simulink model "hw2n_lawB"  (R2022b)
settings: Solver=VariableStepAuto  StartTime=0.0  StopTime=20.0  RelTol=1e-3
undefined symbols (not defined in the file or in its folder): orbit, sat
libraries: matrix_library x1
settings Model: Creator=gagandeepthapar  LastModifiedBy=gagandeepthapar

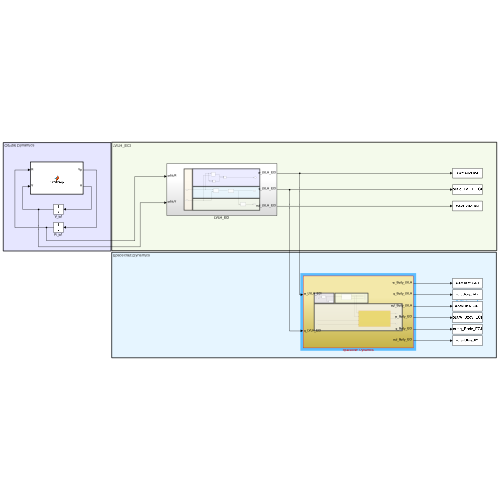
[thumbnail: Simulink's stored preview of the top-level diagram]
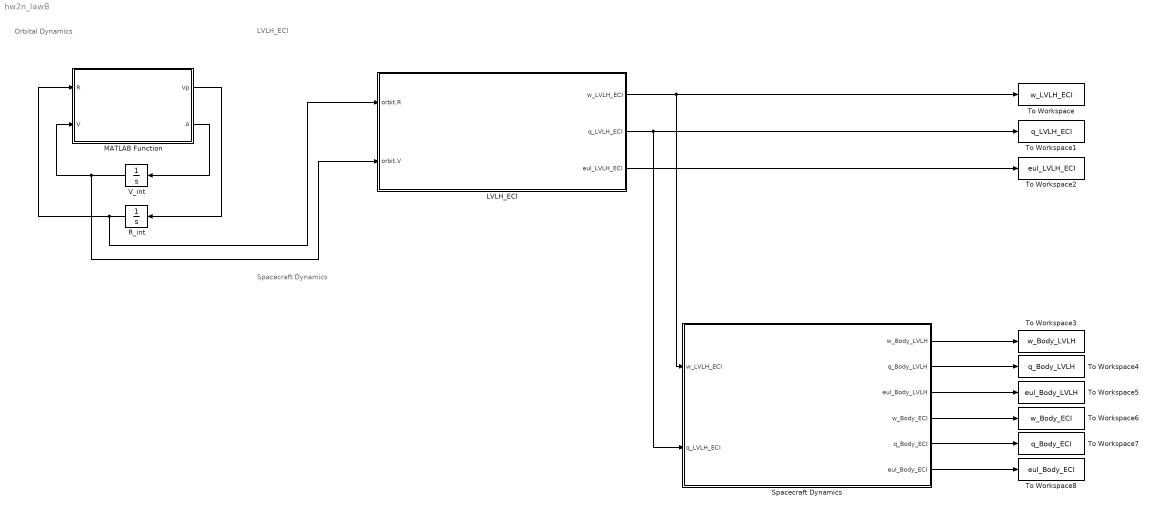
== system hw2n_lawB ==
  note: Spacecraft Dynamics
  note: LVLH_ECI
  note: Orbital Dynamics
  LVLH_ECI : Subsystem
  MATLAB Function : MATLAB Function  TreatAsAtomicUnit=on
  R_int : Integrator  InitialCondition=orbit.R0
  Spacecraft Dynamics : Subsystem
  To Workspace : ToWorkspace  VariableName=w_LVLH_ECI  SampleTime=-1
      settings: Save2DSignal=2-D array (concatenate along first dimension)
  To Workspace1 : ToWorkspace  VariableName=q_LVLH_ECI  SampleTime=-1
      settings: Save2DSignal=2-D array (concatenate along first dimension)
  To Workspace2 : ToWorkspace  VariableName=eul_LVLH_ECI  SampleTime=-1
      settings: Save2DSignal=2-D array (concatenate along first dimension)
  To Workspace3 : ToWorkspace  VariableName=w_Body_LVLH  SampleTime=-1
      settings: Save2DSignal=2-D array (concatenate along first dimension)
  To Workspace4 : ToWorkspace  VariableName=q_Body_LVLH  SampleTime=-1
      settings: Save2DSignal=2-D array (concatenate along first dimension)
  To Workspace5 : ToWorkspace  VariableName=eul_Body_LVLH  SampleTime=-1
      settings: Save2DSignal=2-D array (concatenate along first dimension)
  To Workspace6 : ToWorkspace  VariableName=w_Body_ECI  SampleTime=-1
      settings: Save2DSignal=2-D array (concatenate along first dimension)
  To Workspace7 : ToWorkspace  VariableName=q_Body_ECI  SampleTime=-1
      settings: Save2DSignal=2-D array (concatenate along first dimension)
  To Workspace8 : ToWorkspace  VariableName=eul_Body_ECI  SampleTime=-1
      settings: Save2DSignal=2-D array (concatenate along first dimension)
  V_int : Integrator  InitialCondition=orbit.V0
  wires:
  V_int/1 -> MATLAB Function/2(V), LVLH_ECI/2(orbit.V)
  MATLAB Function/2(A) -> V_int/1
  MATLAB Function/1(Vp) -> R_int/1
  R_int/1 -> MATLAB Function/1(R), LVLH_ECI/1(orbit.R)
  LVLH_ECI/3(eul_LVLH_ECI) -> To Workspace2/1
  LVLH_ECI/1(w_LVLH_ECI) -> To Workspace/1, Spacecraft Dynamics/1(w_LVLH_ECI)
  Spacecraft Dynamics/1(w_Body_LVLH) -> To Workspace3/1
  Spacecraft Dynamics/2(q_Body_LVLH) -> To Workspace4/1
  Spacecraft Dynamics/3(eul_Body_LVLH) -> To Workspace5/1
  Spacecraft Dynamics/5(q_Body_ECI) -> To Workspace7/1
  LVLH_ECI/2(q_LVLH_ECI) -> To Workspace1/1, Spacecraft Dynamics/2(q_LVLH_ECI)
  Spacecraft Dynamics/6(eul_Body_ECI) -> To Workspace8/1
  Spacecraft Dynamics/4(w_Body_ECI) -> To Workspace6/1

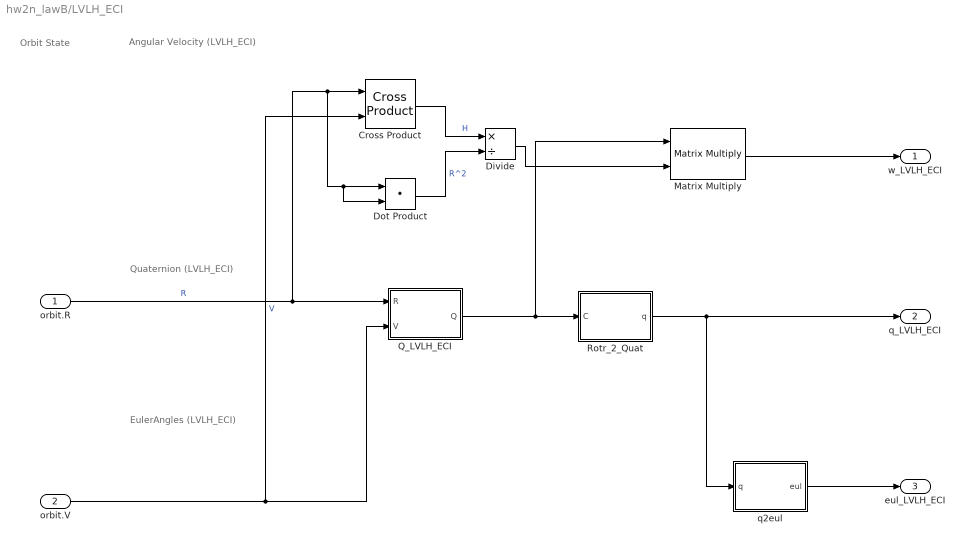
== system hw2n_lawB/LVLH_ECI ==
  note: EulerAngles (LVLH_ECI)
  note: Orbit State
  note: Quaternion (LVLH_ECI)
  note: Angular Velocity (LVLH_ECI)
  orbit.R : Inport
  orbit.V : Inport  Port=2
  Cross Product : matrix_library/Cross Product
  Divide : Product  Inputs=*/
  Dot Product : DotProduct  OutDataTypeStr=Inherit: Inherit via internal rule
  Matrix Multiply : Product  Multiplication=Matrix(*)
  Q_LVLH_ECI : MATLAB Function  TreatAsAtomicUnit=on
  Rotr_2_Quat : MATLAB Function  TreatAsAtomicUnit=on
  q2eul : MATLAB Function  TreatAsAtomicUnit=on
  w_LVLH_ECI : Outport
  q_LVLH_ECI : Outport  Port=2
  eul_LVLH_ECI : Outport  Port=3
  wires:
  orbit.R/1 -> Q_LVLH_ECI/1(R), Cross Product/1, Dot Product/1, Dot Product/2  "R"
  orbit.V/1 -> Cross Product/2, Q_LVLH_ECI/2(V)  "V"
  Q_LVLH_ECI/1(Q) -> Matrix Multiply/1, Rotr_2_Quat/1(C)
  Rotr_2_Quat/1(q) -> q2eul/1(q), q_LVLH_ECI/1
  q2eul/1(eul) -> eul_LVLH_ECI/1
  Cross Product/1 -> Divide/1  "H"
  Dot Product/1 -> Divide/2  "R^2"
  Divide/1 -> Matrix Multiply/2
  Matrix Multiply/1 -> w_LVLH_ECI/1

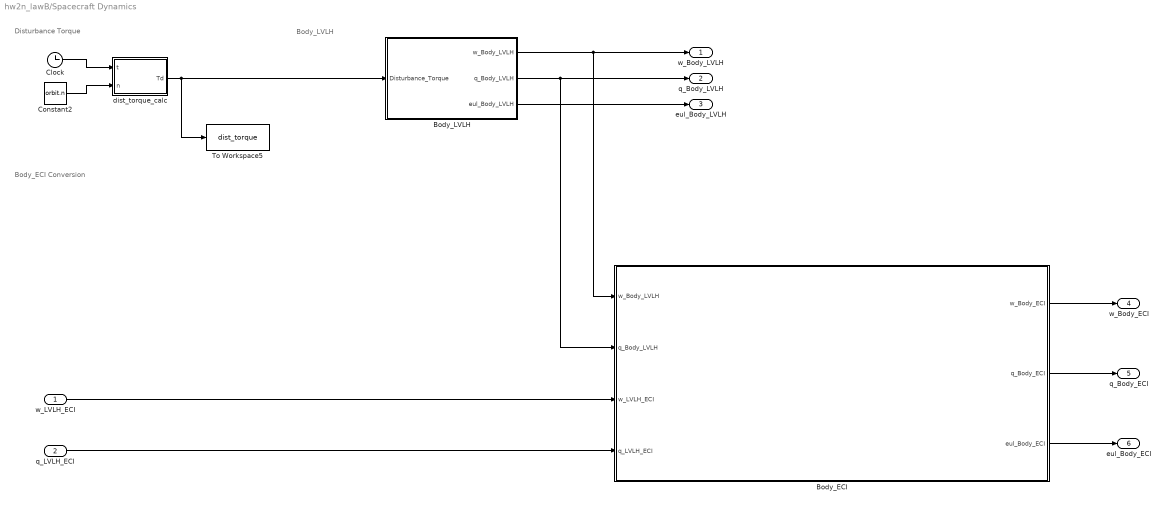
== system hw2n_lawB/Spacecraft Dynamics ==
  note: Body_ECI Conversion
  note: Body_LVLH
  note: Disturbance Torque
  w_LVLH_ECI : Inport
  q_LVLH_ECI : Inport  Port=2
  Body_ECI : Subsystem
  Body_LVLH : Subsystem
  Clock : Clock
  Constant2 : Constant  Value=orbit.n
  To Workspace5 : ToWorkspace  VariableName=dist_torque  SampleTime=-1
      settings: Save2DSignal=2-D array (concatenate along first dimension)
  dist_torque_calc : MATLAB Function  TreatAsAtomicUnit=on
  w_Body_LVLH : Outport
  q_Body_LVLH : Outport  Port=2
  eul_Body_LVLH : Outport  Port=3
  w_Body_ECI : Outport  Port=4
  q_Body_ECI : Outport  Port=5
  eul_Body_ECI : Outport  Port=6
  wires:
  Body_LVLH/1(w_Body_LVLH) -> w_Body_LVLH/1, Body_ECI/1(w_Body_LVLH)
  Body_LVLH/2(q_Body_LVLH) -> Body_ECI/2(q_Body_LVLH), q_Body_LVLH/1
  Body_LVLH/3(eul_Body_LVLH) -> eul_Body_LVLH/1
  Body_ECI/2(q_Body_ECI) -> q_Body_ECI/1
  Constant2/1 -> dist_torque_calc/2(n)
  dist_torque_calc/1(Td) -> Body_LVLH/1(Disturbance_Torque), To Workspace5/1
  Clock/1 -> dist_torque_calc/1(t)
  q_LVLH_ECI/1 -> Body_ECI/4(q_LVLH_ECI)
  w_LVLH_ECI/1 -> Body_ECI/3(w_LVLH_ECI)
  Body_ECI/1(w_Body_ECI) -> w_Body_ECI/1
  Body_ECI/3(eul_Body_ECI) -> eul_Body_ECI/1

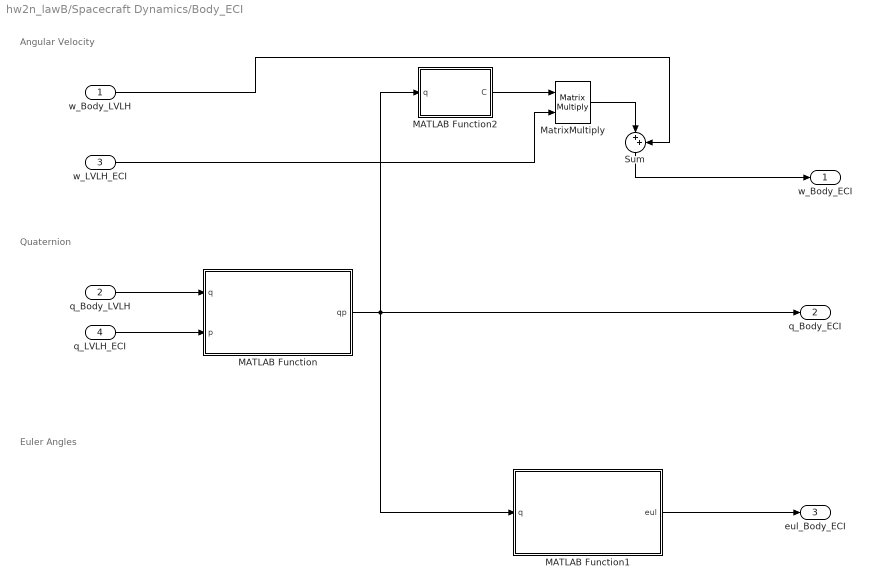
== system hw2n_lawB/Spacecraft Dynamics/Body_ECI ==
  note: Quaternion
  note: Euler Angles
  note: Angular Velocity
  w_Body_LVLH : Inport
  q_Body_LVLH : Inport  Port=2
  w_LVLH_ECI : Inport  Port=3
  q_LVLH_ECI : Inport  Port=4
  MATLAB Function : MATLAB Function  TreatAsAtomicUnit=on
  MATLAB Function1 : MATLAB Function  TreatAsAtomicUnit=on
  MATLAB Function2 : MATLAB Function  TreatAsAtomicUnit=on
  MatrixMultiply : Product  Multiplication=Matrix(*)
  Sum : Sum  Inputs=|++
  w_Body_ECI : Outport
  q_Body_ECI : Outport  Port=2
  eul_Body_ECI : Outport  Port=3
  wires:
  q_Body_LVLH/1 -> MATLAB Function/1(q)
  MATLAB Function/1(qp) -> MATLAB Function2/1(q), MATLAB Function1/1(q), q_Body_ECI/1
  q_LVLH_ECI/1 -> MATLAB Function/2(p)
  MATLAB Function1/1(eul) -> eul_Body_ECI/1
  Sum/1 -> w_Body_ECI/1
  MATLAB Function2/1(C) -> MatrixMultiply/1
  w_LVLH_ECI/1 -> MatrixMultiply/2
  MatrixMultiply/1 -> Sum/1
  w_Body_LVLH/1 -> Sum/2

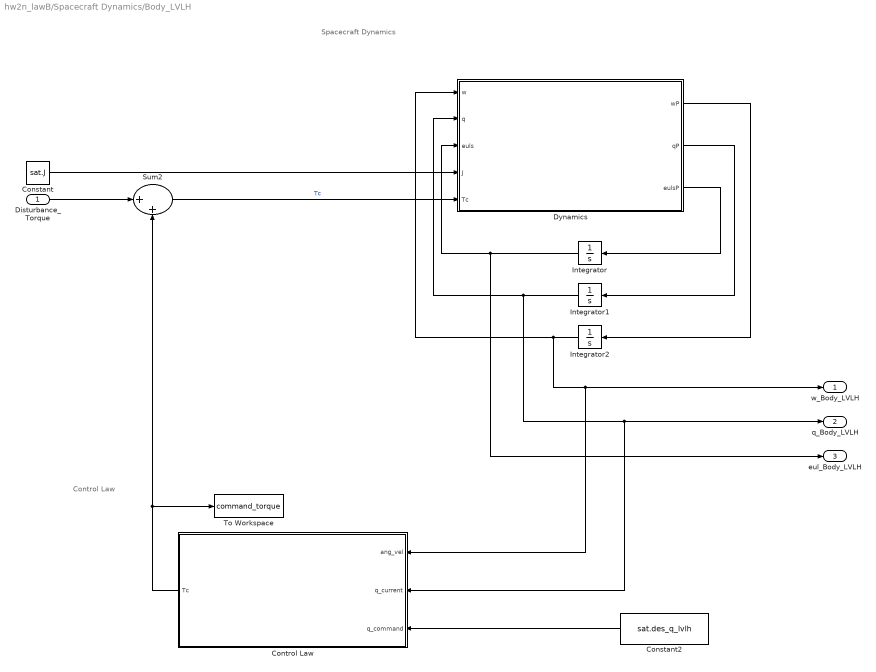
== system hw2n_lawB/Spacecraft Dynamics/Body_LVLH ==
  note: Spacecraft Dynamics
  note: Control Law
  Disturbance_Torque : Inport
  Constant : Constant  Value=sat.J
  Constant2 : Constant  Value=sat.des_q_lvlh
  Control Law : Subsystem
  Dynamics : MATLAB Function  TreatAsAtomicUnit=on
  Integrator : Integrator  InitialCondition=sat.euls0_lvlh
  Integrator1 : Integrator  InitialCondition=[sat.e0_lvlh;sat.n0_lvlh]
  Integrator2 : Integrator  InitialCondition=sat.w0_lvlh
  Sum2 : Sum  Inputs=|++
  To Workspace : ToWorkspace  VariableName=command_torque  SampleTime=-1
      settings: Save2DSignal=2-D array (concatenate along first dimension)
  w_Body_LVLH : Outport
  q_Body_LVLH : Outport  Port=2
  eul_Body_LVLH : Outport  Port=3
  wires:
  Dynamics/3(eulsP) -> Integrator/1
  Dynamics/2(qP) -> Integrator1/1
  Dynamics/1(wP) -> Integrator2/1
  Integrator/1 -> eul_Body_LVLH/1, Dynamics/3(euls)
  Integrator1/1 -> q_Body_LVLH/1, Control Law/2(q_current), Dynamics/2(q)
  Constant/1 -> Dynamics/4(J)
  Disturbance_Torque/1 -> Sum2/1
  Integrator2/1 -> w_Body_LVLH/1, Control Law/1(ang_vel), Dynamics/1(w)
  Sum2/1 -> Dynamics/5(Tc)  "Tc"
  Control Law/1(Tc) -> Sum2/2, To Workspace/1
  Constant2/1 -> Control Law/3(q_command)

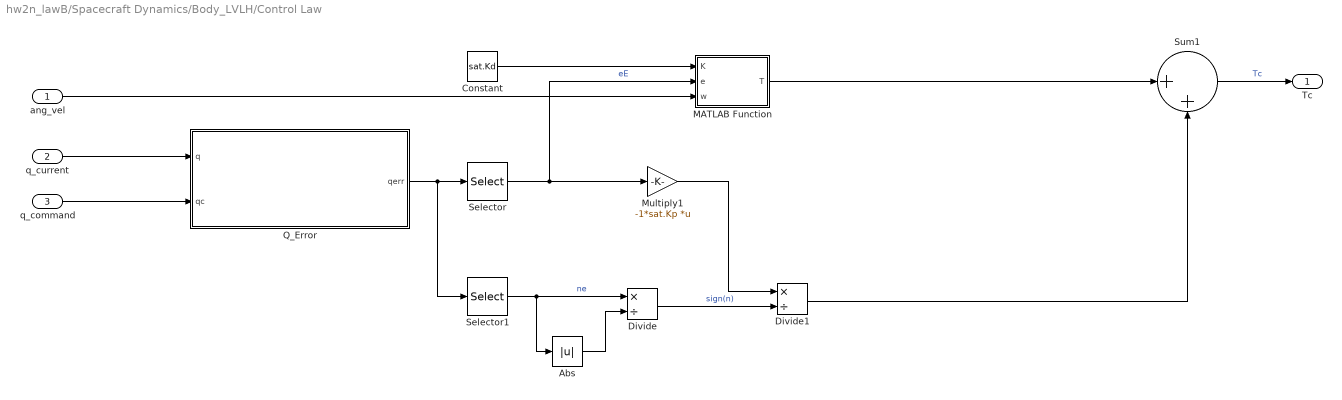
== system hw2n_lawB/Spacecraft Dynamics/Body_LVLH/Control Law ==
  ang_vel : Inport
  q_current : Inport  Port=2
  q_command : Inport  Port=3
  Abs : Abs  SaturateOnIntegerOverflow=off
  Constant : Constant  Value=sat.Kd
  Divide : Product  Inputs=*/
  Divide1 : Product  Inputs=*/
  MATLAB Function : MATLAB Function  TreatAsAtomicUnit=on
  Multiply1 : Gain  Gain=-1*sat.Kp  Multiplication=Matrix(K*u)
  Q_Error : MATLAB Function  TreatAsAtomicUnit=on
  Selector : Selector  InputPortWidth=4  IndexOptions=Index vector (dialog)  Indices=[1:3]  OutputSizes=1
  Selector1 : Selector  InputPortWidth=4  IndexOptions=Index vector (dialog)  Indices=[4]  OutputSizes=1
  Sum1 : Sum  Inputs=|++
  Tc : Outport
  wires:
  Sum1/1 -> Tc/1  "Tc"
  q_command/1 -> Q_Error/2(qc)
  Abs/1 -> Divide/2
  Selector/1 -> MATLAB Function/2(e), Multiply1/1  "eE"
  Divide/1 -> Divide1/2  "sign(n)"
  Selector1/1 -> Divide/1, Abs/1  "ne"
  q_current/1 -> Q_Error/1(q)
  Multiply1/1 -> Divide1/1
  Q_Error/1(qerr) -> Selector/1, Selector1/1
  Divide1/1 -> Sum1/2
  MATLAB Function/1(T) -> Sum1/1
  ang_vel/1 -> MATLAB Function/3(w)
  Constant/1 -> MATLAB Function/1(K)

== matlab function hw2n_lawB/LVLH_ECI/Q_LVLH_ECI ==
  data: R input; Q output; V input
function Q = fcn(R,V)


z = -1*R / norm(R);
y = -1 * cross(R,V) / norm(cross(R,V));

x = cross(y,z);

Q = [x,y,z]';

== matlab function hw2n_lawB/MATLAB Function ==
  data: R input; Vp output; V input; A output
function [Vp,A] = OrbitProp(R,V)

    mu = 398600;

    rad = norm(R);
    rx = R(1);
    ry = R(2);
    rz = R(3);

    ax = -mu*rx/rad^3;
    ay = -mu*ry/rad^3;
    az = -mu*rz/rad^3;

    Vp = [V(1);V(2);V(3)];
    A = [ax;ay;az];

end

== matlab function hw2n_lawB/LVLH_ECI/Rotr_2_Quat ==
  data: C input; q output
function q = fcn(C)

        e = zeros(3,1);
        n = 0.5 * sqrt(1 + trace(C));
        e(1) = 0.25 * (C(2,3) - C(3,2))/n;
        e(2) = 0.25 * (C(3,1) - C(1,3))/n;
        e(3) = 0.25 * (C(1,2) - C(2,1))/n;

        q = [e;n];

== matlab function hw2n_lawB/LVLH_ECI/q2eul ==
  data: q input; eul output
function eul = q2eul(q)

    n = q(4);
    e = q(1:3);

    q = [n, e(1), e(2), e(3)];

    phi = atan2(2*(q(1)*q(2) + q(3)*q(4)), 1 - 2*(q(2)^2 + q(3)^2));
    theta = asin(2*(q(1)*q(3) - q(4)*q(2)));
    psi = atan2(2*(q(1)*q(4) + q(2)*q(3)), 1-2*(q(3)^2 + q(4)^2));

    eul = [phi; theta; psi];

== matlab function hw2n_lawB/Spacecraft Dynamics/Body_LVLH/Dynamics ==
  data: w input; q input; euls input; wP output; J input; Tc input; qP output; eulsP output
function [wP, qP, eulsP] = fcn(w, q, euls, J, Tc)
    
    function wx = skewSymmetric(w)
        wx = [0, -1*w(3), w(2);
             w(3), 0, -1*w(1);
             -1*w(2), w(1), 0];
    end

    T = [Tc(1);Tc(2);Tc(3)];

    wP = J\(T - skewSymmetric(w)*J*w);

    e = q(1:3);
    n = q(4);
    eP = 0.5*(n*eye(3) + skewSymmetric(e))*w;
    nP = -0.5*e'*w;
    qP = [eP;nP];

    phi = euls(1);
    theta = euls(2);
    psi = euls(3);
    eulsP = 1/(cos(theta)) * [cos(theta), sin(phi)*sin(theta), cos(phi)*sin(theta);
                                0, cos(phi)*cos(theta), -1*sin(phi)*cos(theta);
                                0, sin(phi), cos(phi)] * w;


end

== matlab function hw2n_lawB/Spacecraft Dynamics/dist_torque_calc ==
  data: t input; Td output; n input
function Td  = distTorque(t, n)

T = sin(3*n*t)*[0;0.5;0]*10^(-3);
Td = T;
end

== matlab function hw2n_lawB/Spacecraft Dynamics/Body_ECI/MATLAB Function ==
  data: q input; qp output; p input
function qp = quatmult(q, p)
    
        function wx = skewSymmetric(w)
            wx = [0, -1*w(3), w(2);
                 w(3), 0, -1*w(1);
                 -1*w(2), w(1), 0];
        end
    
        qn = q(4);
        qe = q(1:3);
    
        pn = p(4);
        pe = p(1:3);
    
        n = pn * qn - pe'*qe;
        e = pn * qe + qn*pe + skewSymmetric(pe)*qe;
    
        qp = [e(1);e(2);e(3);n];

end

== matlab function hw2n_lawB/Spacecraft Dynamics/Body_LVLH/Control Law/Q_Error ==
  data: q input; qerr output; qc input
function qerr = fcn(q, qc)

%     function wx = skewSymmetric(w)
%         wx = [0, -1*w(3), w(2);
%              w(3), 0, -1*w(1);
%              -1*w(2), w(1), 0];
%     end

    function qp = quatmult(q, p)
    
        function wx = skewSymmetric(w)
            wx = [0, -1*w(3), w(2);
                 w(3), 0, -1*w(1);
                 -1*w(2), w(1), 0];
        end
    
        qn = q(4);
        qe = q(1:3);
    
        pn = p(4);
        pe = p(1:3);
    
        n = pn * qn - pe'*qe;
        e = pn * qe + qn*pe + skewSymmetric(pe)*qe;
    
        qp = [e(1);e(2);e(3);n];
    
    end

qc(1:3) = -1*qc(1:3);
qerr = quatmult(qc, q);

end

== matlab function hw2n_lawB/Spacecraft Dynamics/Body_ECI/MATLAB Function1 ==
  data: q input; eul output
function eul = quat_eul(q)

    n = q(4);
    ex = q(1);
    ey = q(2);
    ez = q(3);

    a = 2*(n*ey - ez*ex);
    if a > 1
        a = 1;
    elseif a < -1
        a = -1;
    end

    phi = atan2(2*(n*ex + ey*ez), 1 - 2*(ex^2 + ey^2));
    theta = asin(a);
    psi = atan2(2*(n*ez + ex*ey), 1 - 2*(ey^2 + ez^2));

    eul = [phi;theta;psi];

end

== matlab function hw2n_lawB/Spacecraft Dynamics/Body_ECI/MATLAB Function2 ==
  data: q input; C output
function C = quat2c(q)

C = quat2rotm([q(4);q(1:3)]');

== matlab function hw2n_lawB/Spacecraft Dynamics/Body_LVLH/Control Law/MATLAB Function ==
  data: K input; T output; e input; w input
function T = fcn(K, e, w)

T = -1*K*(1 - e'*e)*w;
